simulink model "taskBlock_cursorTask_bld"  (R2012b)
settings: Solver=FixedStepDiscrete  StartTime=0.0  StopTime=10.0  FixedStep=0.001  RelTol=1e-3
undefined symbols (not defined in the file): biasCorrectionEnable, biasCorrectionInitial, biasCorrectionPower, biasCorrectionResetToInitial, biasCorrectionStateInds, biasCorrectionTau, biasCorrectionType, biasCorrectionVelocityThreshold, clickHoldTime, clickSource, gloveIndices, gloveThreshold, hmmClickLikelihoodThreshold, hmmClickSpeedMax, hmmResetOnClick, hmmResetOnFast, xkConstants
libraries: xpclib x1
settings Model: Creator=gilja  LastModifiedBy=NPTL
settings SolverCC: EnableConcurrentExecution=on  ConcurrentTasks=on
settings DataIOCC: SaveOutput=off  SignalLogging=off  SaveTime=off
settings OptimizationCC: InlineParams=on  InlineInvariantSignals=on  EnhancedBackFolding=on  EfficientFloat2IntCast=on  SimCompilerOptimization=On
settings DebuggingCC: UnderspecifiedInitializationDetection=Simplified
settings HardwareCC: ProdIntDivRoundTo=Zero  ProdEndianess=LittleEndian  ProdHWDeviceType=Generic->32-bit x86 compatible
settings ModelReferenceCC: ModelReferenceNumInstancesAllowed=Single  ModelReferenceMinAlgLoopOccurrences=on
settings RTWCC: SystemTargetFile=xpctarget.tlc  TemplateMakefile=xpc_default_tmf  Description=xPC Target  ProcessScript=xpctarget_make_rtw_hook  RTWCompilerOptimization=On
settings CodeAppCC: MaxIdLength=62
settings xpcTargetCC: TargetFcnLib=ansi_tfl_table_tmw.mat  CodeReplacementLibrary=XPC_BLAS  ParMdlRefBuildCompliant=on  ConcurrentExecutionCompliant=on  CombineSignalStateStructs=off  GRTInterface=on  xPCTaskExecutionProfile=on  xPCRL32EventNumber=5000  xPCisDownloadable=off  xPCLoadParamSetFile=off  xPCConcurrentTasks=off  xPCEnableSFAnimation=off

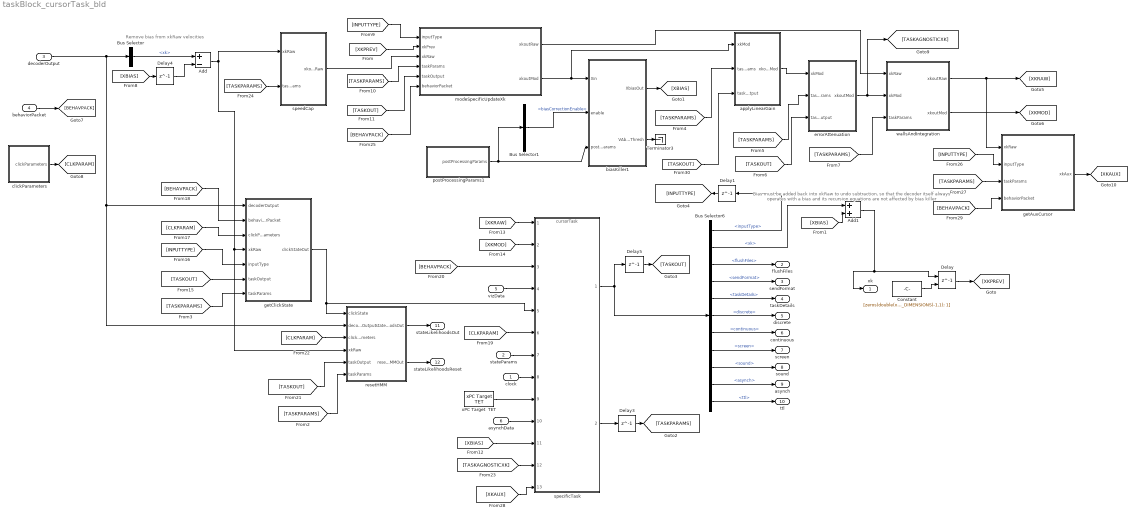
== system taskBlock_cursorTask_bld ==
  note: Remove bias from xkRaw velocities
  note: Bias must be added back into xkRaw to undo subtraction,
      | so that the decoder itself always operates with a bias and its
      | recursion equations are not affected by bias killer
  clock : Inport  OutDataTypeStr=uint32
  stateParams : Inport  Port=2  OutDataTypeStr=Bus: stateParams
  decoderOutput : Inport  Port=3  OutDataTypeStr=Bus: decoderOutput
  behaviorPacket : Inport  Port=4  OutDataTypeStr=Bus: behaviorPacketBus
  vizData : Inport  Port=5  OutDataTypeStr=Bus: peripheralData
  asynchData : Inport  Port=6  OutDataTypeStr=Bus: peripheralData
  Add : Sum  Inputs=+-
  Add1 : Sum
  Bus Selector : BusSelector  OutputSignals=xk
  Bus Selector1 : BusSelector  OutputSignals=biasCorrectionEnable
  Bus Selector6 : BusSelector  OutputSignals=inputType,xk,flushFiles,sendFormat,taskDetails,discrete,continuous,screen,sound,asynch,ttl
  Constant : Constant  Value=[zeros(double(xkConstants.NUM_STATE_DIMENSIONS)-1,1); 1]  VectorParams1D=off
  Delay : Delay  DelayLength=1  InitialConditionSource=Input port  InitialCondition=0
      settings: InputPortMap=u0,p4
  Delay{1,3..5} (4 alike) : Delay  DelayLength=1  InitialCondition=0
  Terminator3 : Terminator
  applyLinearGain : MATLAB Function  TreatAsAtomicUnit=on
  biasKiller1 : MATLAB Function  TreatAsAtomicUnit=on
  clickParameters : Subsystem
  errorAttenuation : MATLAB Function  TreatAsAtomicUnit=on
  getAuxCursor : MATLAB Function  TreatAsAtomicUnit=on
  getClickState : MATLAB Function  TreatAsAtomicUnit=on
  modeSpecificUpdateXk : MATLAB Function  TreatAsAtomicUnit=on
  postProcessingParams1 : Subsystem
  resetHMM : MATLAB Function  TreatAsAtomicUnit=on
  specificTask : ModelReference  ModelNameDialog=cursorTask  SimulationMode=Normal  ModelReferenceVersion=1.2385  CopyOfModelName=cursorTask  DefaultDataLogging=on
  speedCap : MATLAB Function  TreatAsAtomicUnit=on
  wallsAndIntegration : MATLAB Function  TreatAsAtomicUnit=on
  "xPC Target  TET " : xpclib/Misc./xPC Target  TET   ts=0.001
  xk : Outport
  flushFiles : Outport  Port=2
  sendFormat : Outport  Port=3
  taskDetails : Outport  Port=4  OutDataTypeStr=Bus: fileLoggerFormat  BusOutputAsStruct=on
  discrete : Outport  Port=5  OutDataTypeStr=Bus: fileLoggerFormatAndData  BusOutputAsStruct=on
  continuous : Outport  Port=6  OutDataTypeStr=Bus: fileLoggerFormatAndData  BusOutputAsStruct=on
  screen : Outport  Port=7  OutDataTypeStr=Bus: fileLoggerFormatAndData  BusOutputAsStruct=on
  sound : Outport  Port=8  OutDataTypeStr=Bus: fileLoggerFormatAndData  BusOutputAsStruct=on
  asynch : Outport  Port=9  OutDataTypeStr=Bus: fileLoggerFormatAndData  BusOutputAsStruct=on
  ttl : Outport  Port=10  OutDataTypeStr=double  BusOutputAsStruct=on
  stateLikelihoodsOut : Outport  Port=11  OutDataTypeStr=double  BusOutputAsStruct=on
  stateLikelihoodsReset : Outport  Port=12  OutDataTypeStr=double  PortDimensions=1  BusOutputAsStruct=on
  wires:
  specificTask/1 -> Delay5/1, Bus Selector6/1
  Bus Selector6/2 -> Add1/1  "<xk>"
  Bus Selector6/3 -> flushFiles/1  "<flushFiles>"
  Bus Selector6/4 -> sendFormat/1  "<sendFormat>"
  Bus Selector6/6 -> discrete/1  "<discrete>"
  Bus Selector6/7 -> continuous/1  "<continuous>"
  Bus Selector6/5 -> taskDetails/1  "<taskDetails>"
  Bus Selector6/8 -> screen/1  "<screen>"
  Bus Selector6/1 -> Delay1/1  "<inputType>"
  decoderOutput/1 -> resetHMM/2(decoderOutput), getClickState/1(decoderOutput), Bus Selector/1
  Add/1 -> resetHMM/4(xkRaw), getClickState/4(xkRaw), speedCap/1(xkRaw)
  Bus Selector6/11 -> ttl/1  "<ttl>"
  Bus Selector6/9 -> sound/1  "<sound>"
  Bus Selector6/10 -> asynch/1  "<asynch>"
  vizData/1 -> specificTask/4
  resetHMM/1(stateLikelihoodsOut) -> stateLikelihoodsOut/1
  resetHMM/2(resetHMMOut) -> stateLikelihoodsReset/1
  specificTask/2 -> Delay3/1
  asynchData/1 -> specificTask/10
  "xPC Target  TET "/1 -> specificTask/9
  clock/1 -> specificTask/8
  stateParams/1 -> specificTask/7
  Bus Selector/1 -> Add/1  "<xk>"
  Add1/1 -> xk/1, Delay/1
  postProcessingParams1/1(postProcessingParams) -> Bus Selector1/1, biasKiller1/3(postProcParams)
  biasKiller1/2(VAboveThresh) -> Terminator3/1
  Bus Selector1/1 -> biasKiller1/2(enable)  "<biasCorrectionEnable>"
  modeSpecificUpdateXk/2(xkoutMod) -> applyLinearGain/1(xkMod), biasKiller1/1(Xin)
  modeSpecificUpdateXk/1(xkoutRaw) -> wallsAndIntegration/1(xkRaw)
  errorAttenuation/1(xkoutMod) -> [TASKAGNOSTICXK], wallsAndIntegration/2(xkMod)
  Constant/1 -> Delay/2
  Delay/1 -> [XKPREV]
  [XKPREV] -> modeSpecificUpdateXk/2(xkPrev)
  biasKiller1/1(XbiasOut) -> [XBIAS]
  [XBIAS] -> Add1/2
  Delay3/1 -> [TASKPARAMS]
  [TASKPARAMS] -> resetHMM/6(taskParams)
  [TASKPARAMS] -> getClickState/7(taskParams)
  [TASKPARAMS] -> applyLinearGain/2(taskParams)
  [TASKPARAMS] -> errorAttenuation/2(taskParams)
  Delay5/1 -> [TASKOUT]
  [TASKOUT] -> errorAttenuation/3(taskOutput)
  [TASKPARAMS] -> wallsAndIntegration/3(taskParams)
  Delay1/1 -> [INPUTTYPE]
  [INPUTTYPE] -> modeSpecificUpdateXk/1(inputType)
  [XBIAS] -> Delay4/1
  Delay4/1 -> Add/2
  [TASKPARAMS] -> modeSpecificUpdateXk/4(taskParams)
  [TASKOUT] -> modeSpecificUpdateXk/5(taskOutput)
  [XBIAS] -> specificTask/11
  wallsAndIntegration/1(xkoutRaw) -> getAuxCursor/1(xkRaw), [XKRAW]
  wallsAndIntegration/2(xkoutMod) -> [XKMOD]
  [XKRAW] -> specificTask/1
  [XKMOD] -> specificTask/2
  getClickState/1(clickStateOut) -> specificTask/5, resetHMM/1(clickState)
  behaviorPacket/1 -> [BEHAVPACK]
  clickParameters/1(clickParameters) -> [CLKPARAM]
  [TASKOUT] -> getClickState/6(taskOutput)
  [INPUTTYPE] -> getClickState/5(inputType)
  [CLKPARAM] -> getClickState/3(clickParameters)
  [BEHAVPACK] -> getClickState/2(behaviorPacket)
  [CLKPARAM] -> specificTask/6
  [BEHAVPACK] -> specificTask/3
  [TASKOUT] -> resetHMM/5(taskOutput)
  [CLKPARAM] -> resetHMM/3(clickParameters)
  applyLinearGain/1(xkoutMod) -> errorAttenuation/1(xkMod)
  [TASKAGNOSTICXK] -> specificTask/12
  [TASKPARAMS] -> speedCap/2(taskParams)
  speedCap/1(xkoutRaw) -> modeSpecificUpdateXk/3(xkRaw)
  [BEHAVPACK] -> modeSpecificUpdateXk/6(behaviorPacket)
  [INPUTTYPE] -> getAuxCursor/2(inputType)
  [TASKPARAMS] -> getAuxCursor/3(taskParams)
  getAuxCursor/1(xkAux) -> [XKAUX]
  [XKAUX] -> specificTask/13
  [BEHAVPACK] -> getAuxCursor/4(behaviorPacket)
  [TASKOUT] -> applyLinearGain/3(taskOutput)

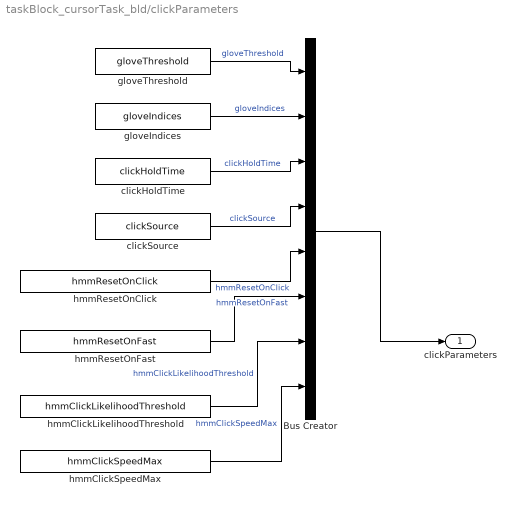
== system taskBlock_cursorTask_bld/clickParameters ==
  Bus Creator : BusCreator  Inputs='gloveThreshold','gloveIndices','clickHoldTime','clickSource','hmmResetOnClick','hmmResetOnFast','hmmClickLikelihoodThreshold','hmmClickSpeedMax'  OutDataTypeStr=Bus: clickParametersBus
  clickHoldTime : Constant  Value=clickHoldTime
  clickSource : Constant  Value=clickSource
  gloveIndices : Constant  Value=gloveIndices
  gloveThreshold : Constant  Value=gloveThreshold
  hmmClickLikelihoodThreshold : Constant  Value=hmmClickLikelihoodThreshold  VectorParams1D=off
  hmmClickSpeedMax : Constant  Value=hmmClickSpeedMax  VectorParams1D=off
  hmmResetOnClick : Constant  Value=hmmResetOnClick  VectorParams1D=off
  hmmResetOnFast : Constant  Value=hmmResetOnFast  VectorParams1D=off
  clickParameters : Outport
  wires:
  Bus Creator/1 -> clickParameters/1
  gloveThreshold/1 -> Bus Creator/1  "gloveThreshold"
  gloveIndices/1 -> Bus Creator/2  "gloveIndices"
  clickHoldTime/1 -> Bus Creator/3  "clickHoldTime"
  clickSource/1 -> Bus Creator/4  "clickSource"
  hmmResetOnClick/1 -> Bus Creator/5  "hmmResetOnClick"
  hmmClickLikelihoodThreshold/1 -> Bus Creator/7  "hmmClickLikelihoodThreshold"
  hmmClickSpeedMax/1 -> Bus Creator/8  "hmmClickSpeedMax"
  hmmResetOnFast/1 -> Bus Creator/6  "hmmResetOnFast"

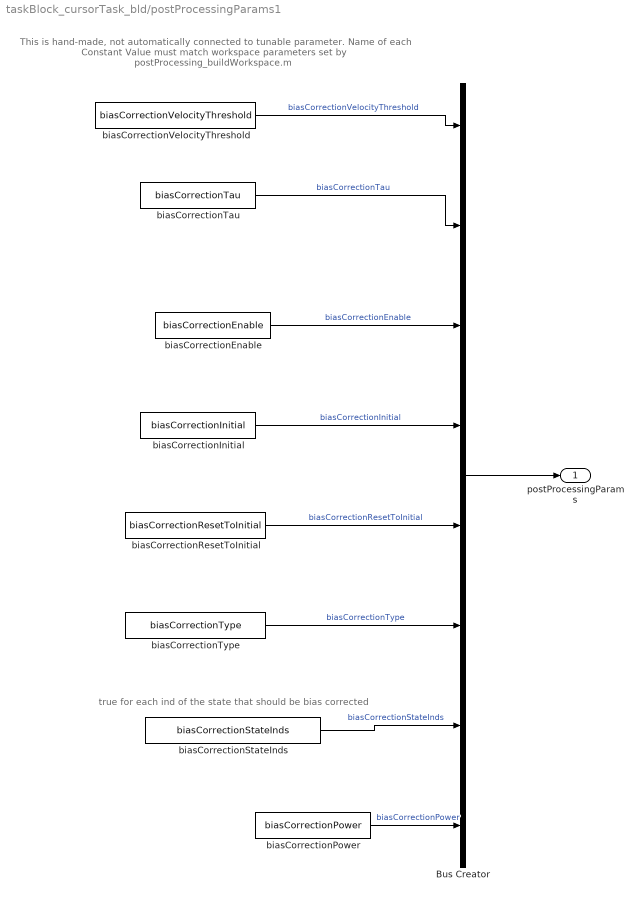
== system taskBlock_cursorTask_bld/postProcessingParams1 ==
  note: true for each ind of the state that should be bias corrected
  note: This is hand-made, not automatically connected to tunable parameter.
      | Name of each Constant Value must match workspace parameters set by
      | postProcessing_buildWorkspace.m
  Bus Creator : BusCreator  Inputs=8  OutDataTypeStr=Bus: postProcessingParams  NonVirtualBus=on
  biasCorrectionEnable : Constant  Value=biasCorrectionEnable
  biasCorrectionInitial : Constant  Value=biasCorrectionInitial
  biasCorrectionPower : Constant  Value=biasCorrectionPower
  biasCorrectionResetToInitial : Constant  Value=biasCorrectionResetToInitial
  biasCorrectionStateInds : Constant  Value=biasCorrectionStateInds
  biasCorrectionTau : Constant  Value=biasCorrectionTau
  biasCorrectionType : Constant  Value=biasCorrectionType
  biasCorrectionVelocityThreshold : Constant  Value=biasCorrectionVelocityThreshold
  postProcessingParams : Outport
  wires:
  Bus Creator/1 -> postProcessingParams/1
  biasCorrectionVelocityThreshold/1 -> Bus Creator/1  "biasCorrectionVelocityThreshold"
  biasCorrectionEnable/1 -> Bus Creator/3  "biasCorrectionEnable"
  biasCorrectionTau/1 -> Bus Creator/2  "biasCorrectionTau"
  biasCorrectionInitial/1 -> Bus Creator/4  "biasCorrectionInitial"
  biasCorrectionResetToInitial/1 -> Bus Creator/5  "biasCorrectionResetToInitial"
  biasCorrectionType/1 -> Bus Creator/6  "biasCorrectionType"
  biasCorrectionStateInds/1 -> Bus Creator/7  "biasCorrectionStateInds"
  biasCorrectionPower/1 -> Bus Creator/8  "biasCorrectionPower"

== matlab function taskBlock_cursorTask_bld/resetHMM ==
  data: clickState input; decoderOutput input Bus: decoderOutput; stateLikelihoodsOut output double; clickParameters input Bus: clickParametersBus; resetHMMOut output; xkRaw input; taskOutput input; taskParams input
function [stateLikelihoodsOut, resetHMMOut] = resetHMM(clickState, decoderOutput, clickParameters, xkRaw, taskOutput, taskParams)
%% takes in all of the state likelihoods and changes move's state likelihood to 1 and the rest to 0 if a reset is triggered
% Checks all the ways the HMM can be reset: 
%%% Exceeding the speed threshold
%%% The click time has elapsed. 
%%% The task says to (eg reset on new trial) 
% only uses the value of clickState to increment the click timer or reset 
%%% SNF warns that the "taskOutput.resetHMM" option doesn't reset the state
%%% likelihoods like the rest of the cases. just so you know. Aug 2019
%%% oh and also the switch statement is uneccessary so if we wanted the
%%% functional bits to be clumped together better, we could just take it
%%% out so it's clear that the clickTime only matters if
%%% clickParameters.hmmResetOnClick is true or the speed crap only gets
%%% calculated if clickParameters.hmmResetOnFast is true. -SNF Anyway,
%%% here's wonderwall. i mean, the code: 
%% define and initialize the persistents 
persistent clickTime; %count how long the click has been held
if isempty(clickTime) %it's the beginning so no clicks yet to count 
    clickTime = 0;
end

persistent prevClickState; %SNF multiclick - compare current click to previous
if isempty(prevClickState) %if there hasn't been a click signal yet, initialize to current clickState
    prevClickState = uint16(clickState); 
end
%% define likelihoods that will be assigned if a reset is triggered
resetLikelihoods = zeros([double(DecoderConstants.MAX_DISCRETE_STATES) 1]); 
resetLikelihoods(1) = 1; % when things are reset, move should be active and no others should be
resetHMMOut = 0; %by default, a reset hasn't been triggered
%% Reset check: has the click exceeded click time? 
%if clickState == uint16(DiscreteStates.CLICK_MAIN) % <- old version, pre-mulitclick
%SNF: increment clickTime if the current click matches the previous one, otherwise reset 
if (uint16(clickState) >= uint16(DiscreteStates.CLICK_MAIN)) % we're currently clicking
    if (prevClickState == uint16(clickState)) || (prevClickState == uint16(DiscreteStates.CLICK_IDLE)) %the previous click was this one OR idle
        clickTime = clickTime+1;
    else %transitioned from a previous click. This shouldn't ever happen but we'll write it out just in case. 
         clickTime = 0; %transitioning from a previous click directly is not allowed, treat it like IDLE  
    end    
else % clickState is IDLE, reset click time
    clickTime = 0;  
end
prevClickState = uint16(clickState); %this should always reflect the last clickState *unless a reset is triggered* (below)
%% copy stateLikelihoods from input to output
stateLikelihoodsOut = decoderOutput.stateLikelihoods;
%% calculate current speed to see if we need to reset bc of speed 
xk2HorizontalVel = uint8( taskParams.xk2HorizontalVel );
xk2VerticalVel   = uint8( taskParams.xk2VerticalVel );
xk2DepthVel      = uint8( taskParams.xk2DepthVel );
velInds          = [xk2HorizontalVel, xk2VerticalVel, xk2DepthVel];
speed            = sqrt(sum(xkRaw(velInds).^2));
%% go through our reset options to see if a reset should be triggered 
switch clickParameters.clickSource %why do we have a switch here? OL never needs this reset so... ? 
    case clickConstants.CLICK_TYPE_NEURAL %Closed loop
    %% we've reach max click time and the task says to auto release after click, reset
        if clickParameters.hmmResetOnClick && clickTime >= clickParameters.clickHoldTime 
            stateLikelihoodsOut = resetLikelihoods; %make move 1 and all others 0
            clickTime = 0;                          %reset the click clock
            resetHMMOut = 1;                        %signal the reset 
            prevClickState = uint16(DiscreteStates.CLICK_IDLE); % update the state
        end
   %% reset to 0 if we're going too fast and the task says to
        if clickParameters.hmmResetOnFast && speed > clickParameters.hmmClickSpeedMax
            stateLikelihoodsOut = resetLikelihoods; %make move 1 and all others 0
            clickTime = 0;                          %reset the click clock
            resetHMMOut = 1;                        %signal the reset 
            prevClickState = uint16(DiscreteStates.CLICK_IDLE); % update the state
        end
   %% task can reset HMM at any time
        if taskOutput.resetHMM %SNF says: WHOAAAAAA WTF why don't we reset the likelihoods here???? But also not touching that. 
            clickTime = 0;
            resetHMMOut = 1;
        end
end %nevermind that this switch statement is useless and is throwing off the groove of the rest of the code.

== matlab function taskBlock_cursorTask_bld/speedCap ==
  data: xkRaw input; xkoutRaw output size=[double(xkConstants.NUM_STATE_DIMENSIONS),1]; taskParams input
function xkoutRaw  = applySpeedCap(xkRaw, taskParams)

%applies speed cap, using the cap in taskParams.xkRawSpeedCap
NUM_DIMS = uint8(cursorConstants.NUM_DIMENSIONS); 
xk2HorizontalVel = uint8( taskParams.xk2HorizontalVel );
xk2VerticalVel = uint8( taskParams.xk2VerticalVel );
xk2DepthVel = uint8( taskParams.xk2DepthVel );
xk2RotateVel = uint8( taskParams.xk2RotateVel );
xk2Rotate2Vel = uint8( taskParams.xk2Rotate2Vel );

canBeVelInds = [xk2HorizontalVel,xk2VerticalVel,xk2DepthVel,xk2RotateVel,xk2Rotate2Vel];
effectorVelInds = canBeVelInds(1:NUM_DIMS);

xkoutRaw = xkRaw;
currentSpeed = sqrt(sum(xkRaw(effectorVelInds).^2)) + eps;
if currentSpeed > taskParams.xkRawSpeedCap
    newSpeed = double(taskParams.xkRawSpeedCap);
else
    newSpeed = currentSpeed;
end
xkoutRaw(effectorVelInds) = xkoutRaw(effectorVelInds) * (newSpeed / currentSpeed);

end

== matlab function taskBlock_cursorTask_bld/biasKiller1 ==
  data: Xin input; enable input; postProcParams input; XbiasOut output; VAboveThresh output
function [XbiasOut, VAboveThresh] = biasKiller(Xin, enable, postProcParams)


speedThreshold = postProcParams.biasCorrectionVelocityThreshold;
tau = postProcParams.biasCorrectionTau;
biasCorrectionInitial = postProcParams.biasCorrectionInitial;
biasCorrectionResetToInitial = postProcParams.biasCorrectionResetToInitial;
biasCorrectionType = postProcParams.biasCorrectionType;
biasCorrectionPower =  postProcParams.biasCorrectionPower; % for BIAS_CORRECTION_SERGEY

% bcInds = postProcParams.biasCorrectionStateInds; % Which elements of state are tracked SDS 7/2016
bcInds = [2:2:20]; %SDS/BJ: should be all the velocity indices of kinematic state

persistent Xbias;
if isempty(Xbias)
    Xbias = zeros(size(Xin));
end
if biasCorrectionResetToInitial
    Xbias = biasCorrectionInitial;
end

VAboveThresh = false;

if enable && tau > 0
    % if tau > 0 update the bias estimate. Setting tau to 0 locks the bias
    % estimate down at whatever it previously was. 
    speed = sqrt( sum( (double(Xin(bcInds))).^2 ) ); %    speed must be greater than some threshold.
 
    switch biasCorrectionType
        % squares each dimension before accumulating it into bias estimate
        case DecoderConstants.BIAS_CORRECTION_FRANK  %% Frank's unbiased killer            
            if (double(speed) > double(speedThreshold))
                Xbias(bcInds) = Xbias(bcInds) + double(Xin(bcInds)) .* abs(double(Xin(bcInds))) ./ double(tau);
                VAboveThresh = true;
            end
            
        case DecoderConstants.BIAS_CORRECTION_BEATA
             % linearly adds each dimension before accumulating it into bias estimate
            if (double(speed) > double(speedThreshold))
                Xbias(bcInds) = Xbias(bcInds) + double(Xin(bcInds)) ./ double(tau);
                VAboveThresh = true;
            end
            
        case DecoderConstants.BIAS_CORRECTION_SERGEY
            % normalizes high-D speed to threshold, then squares, then reverses normalization, then accumulates
            if (double(speed) > double(speedThreshold))                
                normFactor = 1 / double( speedThreshold );
                VinScaled = normFactor .* double( Xin(bcInds) ); % decoded velocity, scaled to >1 by normalizing to speedThreshold
                Vweight = norm( VinScaled ) .^ biasCorrectionPower; % to the power of <biasCorrectionPower> is the scaling rate; so faster speeds weighted  more
                biasUpdate = double(Xin(bcInds)) .* Vweight; % scaled
                biasUpdate = biasUpdate ./ double( tau ); % larger tau slows down bias accumulation.
                Xbias(bcInds) = Xbias(bcInds) + biasUpdate;
                
                VAboveThresh = true;
            end
    end
elseif enable && tau == 0
    % if tau == 0 don't worry about adapting / updating the bias estimate
else
    Xbias = zeros(size(Xin));
end

XbiasOut = Xbias;

== matlab function taskBlock_cursorTask_bld/modeSpecificUpdateXk ==
  data: inputType input uint16 size=1; xkPrev input size=[double(xkConstants.NUM_STATE_DIMENSIONS),1]; xkRaw input size=[double(xkConstants.NUM_STATE_DIMENSIONS),1]; xkoutRaw output size=[double(xkConstants.NUM_STATE_DIMENSIONS),1]; taskParams input; taskOutput input; xkoutMod output size=[double(xkConstants.NUM_STATE_DIMENSIONS),1]; behaviorPacket input
function [xkoutRaw, xkoutMod] = modeSpecificUpdateXk(inputType, xkPrev, xkRaw, taskParams, taskOutput, behaviorPacket)
% xkoutRaw is destined for being fed back into the decoder. 
%xkoutMod ("modified") will affect the task but will not be fed back to the
%decoder. Things like error attenuation should happen to it so that they
%are not compounded by the decoder.

% Most of these persistent variables are used for autoplay (some also for
% error assist). When introducing rotation DOF, I want the autoplay to do
% these rotations *after* the translation. So now there is an additional
% time endpoint (timeFinalRot) 
% -SDS Feb 22 2017
persistent xkStart xTgt prevState timeFinal time timeFinalRot;

NUM_DIMS = uint8(cursorConstants.NUM_DIMENSIONS); % dimensionality of the task. Fixed for a given compile

if(isempty(xkStart))
    xkStart = xkPrev;
    prevState = uint16(0); %% was - uint16(CursorStates.STATE_INIT), this leads to conflicts;
    xTgt = double(zeros(NUM_DIMS,1)); % vector t the target
    timeFinal = 0; % Translation end time.
    timeFinalRot = 0; % Rotation end time. Note that rotation starts after timeFinal + autoplayReactionTime
    time = 0; %will be used to keep track of ti
end

% which state elements do I look to for relevant kinematics pos/vel?
xk2HorizontalPos = uint8( taskParams.xk2HorizontalPos );
xk2VerticalPos = uint8( taskParams.xk2VerticalPos );
xk2HorizontalVel = uint8( taskParams.xk2HorizontalVel );
xk2VerticalVel = uint8( taskParams.xk2VerticalVel );
xk2DepthPos = uint8( taskParams.xk2DepthPos );
xk2DepthVel = uint8( taskParams.xk2DepthVel );
xk2RotatePos = uint8( taskParams.xk2RotatePos );
xk2RotateVel = uint8( taskParams.xk2RotateVel );
xk2Rotate2Pos = uint8( taskParams.xk2Rotate2Pos );
xk2Rotate2Vel = uint8( taskParams.xk2Rotate2Vel );
% DIMENSION-DEPENDENT

canBePosInds = [xk2HorizontalPos,xk2VerticalPos,xk2DepthPos,xk2RotatePos,xk2Rotate2Pos];
effectorPosInds = canBePosInds(1:NUM_DIMS);
canBeVelInds = [xk2HorizontalVel,xk2VerticalVel,xk2DepthVel,xk2RotateVel,xk2Rotate2Vel];
effectorVelInds = canBeVelInds(1:NUM_DIMS);

% Which are translation and which are rotation dimensions?
if NUM_DIMS > 3 % might need to be updated if we add an aperture or other type of DOF later
    NUM_TRANS_DIMS = 3;
    effectorTransPosInds = effectorPosInds(1:NUM_TRANS_DIMS);
    effectorRotPosInds = effectorPosInds(NUM_TRANS_DIMS+1:NUM_DIMS);
    effectorTransVelInds = effectorVelInds(1:NUM_TRANS_DIMS);
    effectorRotVelInds = effectorVelInds(NUM_TRANS_DIMS+1:NUM_DIMS);
    % DIMENSION-DEPENDENT [only if going beyond just rotational dims)
else
    effectorTransPosInds = effectorPosInds;
    effectorRotPosInds = [];
    effectorTransVelInds = effectorVelInds;
    effectorRotVelInds = [];
    NUM_TRANS_DIMS = NUM_DIMS;
end

% SDS October 31 2016
% make last element of xk 1 here. it used to happen in the specificTask,
% which doesn't make sense. Note that we also set this again in the
% decoder, which is redundant, but there it's there just in case we don't
% do it here, and ehre we do it so that this gets logged in
% stream.continuous.xk (since the decoderOutput.xk is different).
xkPrev(end) = 1;

xkoutRaw = xkPrev;

% Set all velocity states to zero. Assumption is that velocity  
% are even indices. These get filled in with modified velocities later in
% this block.
xkoutRaw(2:2:size(xkoutRaw,1)-1) = 0;

% start by making xkoutMod equal to xkoutRaw
xkoutMod = xkoutRaw;

% SDS May 2 2017: Removed logic which checks whether to stop cursor upon a
% click. This is because it was not taking clickHoldTime into account, such
% that a brief click would cause stopping. That's too sensitive.
% Integrating click state to determine selection or velocity zeroing will
% now be relegated to the specificTask.

autoacquireMoveStates = double([CursorStates.STATE_MOVE CursorStates.STATE_MOVE_CLICK CursorStates.STATE_CENTER_TARGET CursorStates.STATE_ACQUIRE CursorStates.STATE_HOVER]);

switch inputType
    case {cursorConstants.INPUT_TYPE_DECODE_V, cursorConstants.INPUT_TYPE_HEAD_CURSORSTILL, ...
            cursorConstants.INPUT_TYPE_CURSOR_HEADSTILL, cursorConstants.INPUT_TYPE_CURSOR_AND_HEAD} 
        % Neural decode -- most common use case
        % Puts this model tick's decoder output into the velocity
        xkoutRaw(effectorVelInds) = xkRaw(effectorVelInds);
        xkoutMod(effectorVelInds) = xkRaw(effectorVelInds);
        
        % Nonlinear gain.
        % applies a nonlinear power gain, which is governed by
        % two parameters. the powerGain determines the shape
        % of the curve (higher values have a steeper rise).
        % The powerGainUnityCrossing defines the superlinear cross-over point
        % after which the output equals the input. - SDS April 2017
        inSpeed = sqrt( sum(  xkoutMod(effectorVelInds).^2 ) );
        inScaled =  inSpeed./ taskParams.powerGainUnityCrossing; % speed, as a multiple of unity crossing
        outScaled = inScaled ^ taskParams.powerGain; % how much slower/faster it got
        if inSpeed < eps
            % avoids nans when divide by 0 would happen
            unitNormVel =  xkoutMod(effectorVelInds);
        else
            unitNormVel =  xkoutMod(effectorVelInds) ./ inSpeed;
        end
        xkoutMod(effectorVelInds) = (outScaled*taskParams.powerGainUnityCrossing) .* unitNormVel;

    case {cursorConstants.INPUT_TYPE_AUTO_ACQUIRE, cursorConstants.INPUT_TYPE_AUTO_ACQUIRE_HS, cursorConstants.INPUT_TYPE_WIA_HEAD} % ASSUMES CENTER OUT (AND BACK) WITH A SINGLE FIXED TGT DISTANCE
        if( ((prevState ~= CursorStates.STATE_MOVE) && (taskOutput.state == CursorStates.STATE_MOVE)) ...
                || ((prevState ~= CursorStates.STATE_MOVE_CLICK) && (taskOutput.state == CursorStates.STATE_MOVE_CLICK)) ...
                || ((prevState ~= CursorStates.STATE_CENTER_TARGET) && taskOutput.state == CursorStates.STATE_CENTER_TARGET))
            % game just entered one of the autoplay states, so compute
            % the vector towards the target and how long it should take
            % to get there.
            xkStart = xkPrev;
            xTgt = double(taskOutput.currentTarget(1:NUM_DIMS)) - ...
                double(xkPrev(effectorPosInds));
            
            % When translation ends: 1 autoplayReactionTime added
            if taskOutput.wiaCode==1
                speedMultiplier = 1;
                if taskOutput.speedCode==1
                    speedMultiplier = 3;
                elseif taskOutput.speedCode==2
                    speedMultiplier = 1.5;
                elseif taskOutput.speedCode==3
                    speedMultiplier = 0.75;
                end
                timeMultiplier = speedMultiplier * log(sqrt(sum(xTgt.^2)))/6.0137;
            else
                timeMultiplier = 1;
            end
            
            timeFinal = round( timeMultiplier * double( taskParams.autoplayReactionTime + taskParams.autoplayMovementDuration ) );
            
            % When rotation ends: it starts 1
            % autoplayReactionTime *after* translation ends
            timeFinalRot = round( double( taskParams.autoplayRotationStart + taskParams.autoplayRotationDuration ) );
            
            time = 0;
        elseif any(double(taskOutput.state) == autoacquireMoveStates)
            % what fraction of the translation is complete (from 0
            % to 1):
            transStartsAt = double( taskParams.autoplayReactionTime );
            tau = min( max(0, time - transStartsAt)/(timeFinal-transStartsAt), 1); % this is what it was before I fixed this on July 12 2017 -SDS
            
            % What fraction of the rotation is complete( from 0 to
            % 1)
            rotStartsAt = double( taskParams.autoplayRotationStart);
            tauRot = min( max(0, time - rotStartsAt)/(timeFinalRot-rotStartsAt) , 1); 
            
            % do this to both raw and modified. I'm not sure if we
            % actually do anything with the raw xk during filter
            % building but might as well keep behavior consistent
            % with how it was before we separated xkoutRaw and
            % xkoutMod.
            % Old way, before breaking out translation and rotation
            %                     xkoutRaw(effectorPosInds) = xkStart(effectorPosInds(1:NUM_DIMS)) -  xTgt(1:NUM_DIMS)* double( (15*tau^4 - 6*tau^5 - 10*tau^3) ); % 1:NUM_DIMS to handhold compiler
            %                     xkoutRaw(effectorVelInds) = xkoutRaw(effectorPosInds) - xkPrev(effectorPosInds);
            %                     xkoutMod(effectorPosInds) = xkoutRaw(effectorPosInds);
            %                     xkoutMod(effectorVelInds) = xkoutRaw(effectorVelInds);
            % TRANSLATION
            xkoutRaw(effectorTransPosInds) = xkStart(effectorTransPosInds) -  xTgt(1:NUM_TRANS_DIMS)* double( (15*tau^4 - 6*tau^5 - 10*tau^3) );
            xkoutRaw(effectorTransVelInds) = xkoutRaw(effectorTransPosInds) - xkPrev(effectorTransPosInds);
            xkoutMod(effectorTransPosInds) = xkoutRaw(effectorTransPosInds);
            xkoutMod(effectorTransVelInds) = xkoutRaw(effectorTransVelInds);
            
            % ROTATION
            xkoutRaw(effectorRotPosInds) = xkStart(effectorRotPosInds) -  xTgt(NUM_TRANS_DIMS+1:NUM_DIMS)* double( (15*tauRot^4 - 6*tauRot^5 - 10*tauRot^3) );
            xkoutRaw(effectorRotVelInds) = xkoutRaw(effectorRotPosInds) - xkPrev(effectorRotPosInds);
            xkoutMod(effectorRotPosInds) = xkoutRaw(effectorRotPosInds);
            xkoutMod(effectorRotVelInds) = xkoutRaw(effectorRotVelInds);
            
            time = time + 1; % time since this autoplay began counts up..
        else
            xkoutRaw(effectorVelInds) = 0;
            xkoutMod(effectorVelInds) = 0;
        end
        
    case cursorConstants.INPUT_TYPE_NONE
        xkoutRaw(effectorVelInds) = 0;
        xkoutMod(effectorVelInds) = 0;
        
    case cursorConstants.INPUT_TYPE_HEAD_MOUSE
        xkoutRaw(effectorPosInds(1)) = behaviorPacket.windowsMousePosition(1)*1080;
        xkoutRaw(effectorPosInds(2)) = -behaviorPacket.windowsMousePosition(2)*1080;
        
        xkoutMod(effectorPosInds(1)) = behaviorPacket.windowsMousePosition(1)*1080;
        xkoutMod(effectorPosInds(2)) = -behaviorPacket.windowsMousePosition(2)*1080;
        
        R = [cosd(taskParams.vmrTheta), -sind(taskParams.vmrTheta); sind(taskParams.vmrTheta), cosd(taskParams.vmrTheta)]; 
        xkoutMod(effectorPosInds(1:2)) = R*xkoutMod(effectorPosInds(1:2));
        
        xkoutRaw(effectorVelInds) = 0;
        xkoutMod(effectorVelInds) = 0;
        
    otherwise
        xkoutRaw(effectorVelInds) = 0;
        xkoutMod(effectorVelInds) = 0;
end

%for autoplay
prevState = uint16(taskOutput.state);

end

== matlab function taskBlock_cursorTask_bld/applyLinearGain ==
  data: xkMod input; xkoutMod output size=[double(xkConstants.NUM_STATE_DIMENSIONS),1]; taskParams input; taskOutput input
function xkoutMod  = applyLinearGain(xkMod, taskParams, taskOutput)

%applies linear gains to each dimension as specified in taskParams
NUM_DIMS = uint8(cursorConstants.NUM_DIMENSIONS); 
xk2HorizontalVel = uint8( taskParams.xk2HorizontalVel );
xk2VerticalVel = uint8( taskParams.xk2VerticalVel );
xk2DepthVel = uint8( taskParams.xk2DepthVel );
xk2RotateVel = uint8( taskParams.xk2RotateVel );
xk2Rotate2Vel = uint8( taskParams.xk2Rotate2Vel );

canBeVelInds = [xk2HorizontalVel,xk2VerticalVel,xk2DepthVel,xk2RotateVel,xk2Rotate2Vel];
effectorVelInds = canBeVelInds(1:NUM_DIMS);

xkoutMod = xkMod;
xkoutMod(effectorVelInds) = xkMod(effectorVelInds) .* taskParams.gain(1:NUM_DIMS,1);
if uint16(taskOutput.state) == CursorStates.STATE_NEW_TARGET
    xkoutMod(effectorVelInds) = xkoutMod(effectorVelInds) .* taskParams.delayPeriodGainScale;
end
end

== matlab function taskBlock_cursorTask_bld/wallsAndIntegration ==
  data: xkRaw input; xkMod input size=[double(xkConstants.NUM_STATE_DIMENSIONS),1]; xkoutRaw output size=[double(xkConstants.NUM_STATE_DIMENSIONS),1]; taskParams input; xkoutMod output size=[double(xkConstants.NUM_STATE_DIMENSIONS),1]
function [xkoutRaw, xkoutMod] = wallsAndIntegration(xkRaw, xkMod, taskParams)
% xkoutRaw is destined for being fed back into the decoder. 
%xkoutMod ("modified") will affect the task but will not be fed back to the
%decoder. Things like error attenuation should happen to it so that they
%are not compounded by the decoder.

NUM_DIMS = uint8(cursorConstants.NUM_DIMENSIONS); % dimensionality of the task. Fixed for a given compile

% which state elements do I look to for relevant kinematics pos/vel?
xk2HorizontalPos = uint8( taskParams.xk2HorizontalPos );
xk2VerticalPos = uint8( taskParams.xk2VerticalPos );
xk2HorizontalVel = uint8( taskParams.xk2HorizontalVel );
xk2VerticalVel = uint8( taskParams.xk2VerticalVel );
xk2DepthPos = uint8( taskParams.xk2DepthPos );
xk2DepthVel = uint8( taskParams.xk2DepthVel );
xk2RotatePos = uint8( taskParams.xk2RotatePos );
xk2RotateVel = uint8( taskParams.xk2RotateVel );
xk2Rotate2Pos = uint8( taskParams.xk2Rotate2Pos );
xk2Rotate2Vel = uint8( taskParams.xk2Rotate2Vel );

canBePosInds = [xk2HorizontalPos,xk2VerticalPos,xk2DepthPos,xk2RotatePos,xk2Rotate2Pos];
effectorPosInds = canBePosInds(1:NUM_DIMS);
canBeVelInds = [xk2HorizontalVel,xk2VerticalVel,xk2DepthVel,xk2RotateVel,xk2Rotate2Vel];
effectorVelInds = canBeVelInds(1:NUM_DIMS);

xkoutRaw = xkRaw;
xkoutMod = xkMod;

%% integrates velocity into change of position (important, obviously)
%R = [cosd(taskParams.vmrTheta), -sind(taskParams.vmrTheta); sind(taskParams.vmrTheta), cosd(taskParams.vmrTheta)]; 
%xkoutMod(effectorVelInds(1:2)) = R*xkoutMod(effectorVelInds(1:2));
 
xkoutRaw(effectorPosInds) = xkoutRaw(effectorPosInds) + xkoutRaw(effectorVelInds);
xkoutMod(effectorPosInds) = xkoutMod(effectorPosInds) + xkoutMod(effectorVelInds);

%% Boundaries to workspace
% Horizontal
if xkoutMod(taskParams.xk2HorizontalPos) > taskParams.workspaceX(2)
    xkoutMod(taskParams.xk2HorizontalPos) = taskParams.workspaceX(2);
    xkoutMod(taskParams.xk2HorizontalVel) = 0;
elseif xkoutMod(taskParams.xk2HorizontalPos) < taskParams.workspaceX(1)
    xkoutMod(taskParams.xk2HorizontalPos) = taskParams.workspaceX(1);
    xkoutMod(taskParams.xk2HorizontalVel) = 0;
end
% Vertical
if xkoutMod(taskParams.xk2VerticalPos) > taskParams.workspaceY(2)
    xkoutMod(taskParams.xk2VerticalPos) = taskParams.workspaceY(2);
    xkoutMod(taskParams.xk2VerticalVel) = 0;
elseif xkoutMod(taskParams.xk2VerticalPos) < taskParams.workspaceY(1)
    xkoutMod(taskParams.xk2VerticalPos) = taskParams.workspaceY(1);
    xkoutMod(taskParams.xk2VerticalVel) = 0;
end
% Depth
if xkoutMod(taskParams.xk2DepthPos) > taskParams.workspaceZ(2)
    xkoutMod(taskParams.xk2DepthPos) = taskParams.workspaceZ(2);
    xkoutMod(taskParams.xk2DepthVel) = 0;
elseif xkoutMod(taskParams.xk2DepthPos) < taskParams.workspaceZ(1)
    xkoutMod(taskParams.xk2DepthPos) = taskParams.workspaceZ(1);
    xkoutMod(taskParams.xk2DepthVel) = 0;
end
% Rotate 1 (around the Z axis)
if xkoutMod(taskParams.xk2RotatePos) > taskParams.workspaceR(2)
    xkoutMod(taskParams.xk2RotatePos) = taskParams.workspaceR(2);
    xkoutMod(taskParams.xk2RotateVel) = 0;
elseif xkoutMod(taskParams.xk2RotatePos) < taskParams.workspaceR(1)
    xkoutMod(taskParams.xk2RotatePos) = taskParams.workspaceR(1);
    xkoutMod(taskParams.xk2RotateVel) = 0;
end
% Rotate 2 (around the Y axis)
if xkoutMod(taskParams.xk2Rotate2Pos) > taskParams.workspaceR2(2)
    xkoutMod(taskParams.xk2Rotate2Pos) = taskParams.workspaceR2(2);
    xkoutMod(taskParams.xk2Rotate2Vel) = 0;
elseif xkoutMod(taskParams.xk2Rotate2Pos) < taskParams.workspaceR2(1)
    xkoutMod(taskParams.xk2Rotate2Pos) = taskParams.workspaceR2(1);
    xkoutMod(taskParams.xk2Rotate2Vel) = 0;
end

% DIMENSION-DEPENDENT
% xkoutRaw's positions should always match xkoutMod's positions, so
% decoder knows displayed cursor position.
xkoutRaw(effectorPosInds) =  xkoutMod(effectorPosInds);

end

== matlab function taskBlock_cursorTask_bld/errorAttenuation ==
  data: xkMod input; taskParams input; taskOutput input; xkoutMod output size=[double(xkConstants.NUM_STATE_DIMENSIONS),1]
function xkoutMod   = errorAttenuation(xkMod, taskParams, taskOutput)
% xkoutRaw is destined for being fed back into the decoder. 
%xkoutMod ("modified") will affect the task but will not be fed back to the
%decoder. Things like error attenuation should happen to it so that they
%are not compounded by the decoder.

% Most of these persistent variables are used for autoplay (some also for
% error assist). When introducing rotation DOF, I want the autoplay to do
% these rotations *after* the translation. So now there is an additional
% time endpoint (timeFinalRot) 
% -SDS Feb 22 2017

NUM_DIMS = uint8(cursorConstants.NUM_DIMENSIONS); % dimensionality of the task. Fixed for a given compile

% which state elements do I look to for relevant kinematics pos/vel?
xk2HorizontalPos = uint8( taskParams.xk2HorizontalPos );
xk2VerticalPos = uint8( taskParams.xk2VerticalPos );
xk2HorizontalVel = uint8( taskParams.xk2HorizontalVel );
xk2VerticalVel = uint8( taskParams.xk2VerticalVel );
xk2DepthPos = uint8( taskParams.xk2DepthPos );
xk2DepthVel = uint8( taskParams.xk2DepthVel );
xk2RotatePos = uint8( taskParams.xk2RotatePos );
xk2RotateVel = uint8( taskParams.xk2RotateVel );
xk2Rotate2Pos = uint8( taskParams.xk2Rotate2Pos );
xk2Rotate2Vel = uint8( taskParams.xk2Rotate2Vel );

canBePosInds = [xk2HorizontalPos,xk2VerticalPos,xk2DepthPos,xk2RotatePos,xk2Rotate2Pos];
effectorPosInds = canBePosInds(1:NUM_DIMS);
canBeVelInds = [xk2HorizontalVel,xk2VerticalVel,xk2DepthVel,xk2RotateVel,xk2Rotate2Vel];
effectorVelInds = canBeVelInds(1:NUM_DIMS);

%% apply assist if specified in taskParams
% only apply when task is unpaused
xkoutMod = xkMod;
if isfield(taskParams,'errorAssistTheta') && ~taskOutput.paused % because some tasks might not have error assist
    errorAssistTheta = double( taskParams.errorAssistTheta(1:NUM_DIMS) );     %BJ: should now be a vector (one value for each dimension in NUM_DIMS)
    errorAssistR = double( taskParams.errorAssistR(1:NUM_DIMS) );             %BJ: should now be a vector (one value for each dimension in NUM_DIMS)
    errorAssistAxis = double( taskParams.errorAssistAxis(1:NUM_DIMS) );          %Added by SDS Oct 2016
    
    % start with modified xk, which may have had gain applied to it.
    xkVel = xkoutMod(effectorVelInds);                             %BJ: current decoded cursor velocity
    xT = double(taskOutput.currentTarget(1:NUM_DIMS)) - double(xkMod(effectorPosInds)); %BJ: cursor pos to target pos vector
    
    if sum( abs(xT) < 0.001 ) == NUM_DIMS   %BJ: if cursor is within 1 mm of target in every dimension,
        %skip rest of steps in EA, rather than error-assisting
    else
        %BJ: apply error assist
        xNormT = xT ./ sqrt(sum(xT.^2));    %BJ: xNormT is normalized xT, points towards target
        projT_sc = dot(xkVel, xNormT);        %BJ: scalar projection of xkVel on xT
        projT = double( zeros( 1, NUM_DIMS ) ); % initialize
        squashVelFactor = double( zeros( 1, NUM_DIMS ) ); % initialize
        
        %BJ: apply magnitude (Rho) assist only if projection is negative
        if projT_sc < 0 % if decoded velocity was poiting away from target...
            % ... Reduce the speed according to errorAssistR, up to
            % just not allowing any movement.
            projT = projT_sc*(1-errorAssistR);   %BJ: changes the projT that gets added to the decoded velocity...
            squashVelFactor = 1 - errorAssistR;     %... and squashes the output velocity if going in wrong direction
        else
            % This happens if we're headed towards target
            projT(1:NUM_DIMS) = projT_sc;   %BJ: still need to copy projT_sc into each dimension
            squashVelFactor(1:NUM_DIMS) = 1;            %BJ: leave velocity the same
        end
        % apply error correction to modified xk
        xkoutMod(effectorVelInds) = projT.*errorAssistTheta.*xNormT' + squashVelFactor.*(1 - errorAssistTheta).*xkVel';
        
        % errorAssistAxis operates last. This will reduce the velocity
        % along every cardinal axis between 0 and 1 if and only if the
        % velocity along this axis is away from the target's coordinate
        % This looks at the final velocity *after* errorAssistTheta and
        % errorAssistR were used. Though, honestly, I haven't thought
        % through the case when one would use both errorAssistR and
        % check which
        modDims = sign(xkoutMod(effectorVelInds).*xT) < 0; % 1s for any axis it's moving the wrong way at.
        % errorAssistAxis == 0 means do nothing, hence 1-__
        xkoutMod(effectorVelInds(modDims)) = xkoutMod(effectorVelInds(modDims)).*(1-errorAssistAxis(modDims))';
    end
end

end

== matlab function taskBlock_cursorTask_bld/getAuxCursor ==
  data: xkRaw input; inputType input; xkAux output size=[double(xkConstants.NUM_STATE_DIMENSIONS),1]; taskParams input; behaviorPacket input
function xkAux = getAuxCursor(xkRaw, inputType, taskParams, behaviorPacket)
    %Some modes have an extra "auxiliary" cursor (e.g. when the head mouse cursor must be
    %held still while the BCI cursor must acquire targets as normal). Based on the mode, this block
    %outputs the auxiliary cursor state. Right now it works only for the head
    %mouse. 

    NUM_DIMS = uint8(cursorConstants.NUM_DIMENSIONS); 

    xk2HorizontalPos = uint8( taskParams.xk2HorizontalPos );
    xk2VerticalPos = uint8( taskParams.xk2VerticalPos );
    xk2HorizontalVel = uint8( taskParams.xk2HorizontalVel );
    xk2VerticalVel = uint8( taskParams.xk2VerticalVel );
    xk2DepthPos = uint8( taskParams.xk2DepthPos );
    xk2DepthVel = uint8( taskParams.xk2DepthVel );
    xk2RotatePos = uint8( taskParams.xk2RotatePos );
    xk2RotateVel = uint8( taskParams.xk2RotateVel );
    xk2Rotate2Pos = uint8( taskParams.xk2Rotate2Pos );
    xk2Rotate2Vel = uint8( taskParams.xk2Rotate2Vel );

    canBePosInds = [xk2HorizontalPos,xk2VerticalPos,xk2DepthPos,xk2RotatePos,xk2Rotate2Pos];
    effectorPosInds = canBePosInds(1:NUM_DIMS);
    canBeVelInds = [xk2HorizontalVel,xk2VerticalVel,xk2DepthVel,xk2RotateVel,xk2Rotate2Vel];
    effectorVelInds = canBeVelInds(1:NUM_DIMS);

    xkAux = zeros(size(xkRaw));

    switch inputType
        case {cursorConstants.INPUT_TYPE_HEAD_CURSORSTILL, cursorConstants.INPUT_TYPE_CURSOR_HEADSTILL, ...
                cursorConstants.INPUT_TYPE_AUTO_ACQUIRE_HS, cursorConstants.INPUT_TYPE_CURSOR_AND_HEAD, cursorConstants.INPUT_TYPE_WIA_HEAD}
            xkAux(effectorPosInds(1)) = behaviorPacket.windowsMousePosition(1)*1080;
            xkAux(effectorPosInds(2)) = -behaviorPacket.windowsMousePosition(2)*1080;
            xkAux(effectorVelInds) = 0;

        otherwise
            xkAux(effectorVelInds) = 0;
            xkAux(effectorVelInds) = 0; 
    end
end

== matlab function taskBlock_cursorTask_bld/getClickState ==
  data: decoderOutput input; behaviorPacket input Bus: behaviorPacketBus; clickStateOut output uint16; clickParameters input Bus: clickParametersBus; xkRaw input; inputType input; taskOutput input; taskParams input
function clickStateOut = getClickState(decoderOutput, behaviorPacket, clickParameters, xkRaw, inputType, taskOutput, taskParams)
% clickStateOut ranges from IDLE to any of the clicks (multiclick) -
% identify it based on the state likelihoods in decoderOutput and
% clickParameters (for the threshold). This block takes the decoded output
% and does the deciding so the task only gets the decoded click value. 
% -last modified and commented by SNF, August 2019 
% the xk here is xkRaw 
%% define the (unecessary) persistent. SNF can't spell unnecessary and she knows. uneccessary? *shrugs*
% SNF: this initialization is uneccessary, also doesn't need to be persistent since we
% always set it to idle at the beginning.... 
%  persistent clickState ;
% if isempty(clickState)
%     clickState = uint16(DiscreteStates.CLICK_IDLE);
% end
clickState = uint16(DiscreteStates.CLICK_IDLE); %SNF: this line was already here, outside of the if so yeah no persistence necessary
%% get the cursor position (- but really the velocity is all that matters -SNF) 
% which state elements do I look to for the cursor's position? SDS July 2016
NUM_DIMS         = uint8(cursorConstants.NUM_DIMENSIONS); % 
xk2HorizontalPos = uint8( taskParams.xk2HorizontalPos );
xk2VerticalPos   = uint8( taskParams.xk2VerticalPos );
xk2HorizontalVel = uint8( taskParams.xk2HorizontalVel );
xk2VerticalVel   = uint8( taskParams.xk2VerticalVel );
xk2DepthPos      = uint8( taskParams.xk2DepthPos );
xk2DepthVel      = uint8( taskParams.xk2DepthVel );
xk2RotatePos     = uint8( taskParams.xk2RotatePos );
xk2RotateVel     = uint8( taskParams.xk2RotateVel );
xk2Rotate2Pos    = uint8( taskParams.xk2Rotate2Pos );
xk2Rotate2Vel    = uint8( taskParams.xk2Rotate2Vel );
% TASK_DIMS = taskParams.numDisplayDims; % only used for determining what kind of
% % checking to use. We still need to have everything be NUM_DIMS long or things won't compile.
canBePosInds = [xk2HorizontalPos,xk2VerticalPos,xk2DepthPos,xk2RotatePos,xk2Rotate2Pos];
canBeVelInds = [xk2HorizontalVel,xk2VerticalVel,xk2DepthVel,xk2RotateVel,xk2Rotate2Vel];
effectorPosInds = canBePosInds(1:NUM_DIMS);
effectorVelInds = canBeVelInds(1:NUM_DIMS);
% and get the speed while we're here
speed = sqrt(sum(xkRaw(effectorVelInds).^2));
%% initialize multiclick variables 
CLICK_INDICES = 2: uint16(DecoderConstants.MAX_DISCRETE_STATES);
maxCS  = double(0); % there is some CRAZY type casting necessary for Simulink, don't mind this.... 
maxL   = double(0);
%% handle ancient artifacts: 
gloveData = behaviorPacket.glove;
if behaviorPacket.gloveSerial2(6) == 'L'
    gloveData = behaviorPacket.glove2;
end
% less ancient, still old and unused: 
mouseData = behaviorPacket.mouse;
%% assign clickState values!
if inputType == cursorConstants.INPUT_TYPE_AUTO_ACQUIRE % OL is so easy 
    if taskOutput.state == CursorStates.STATE_HOVER     % if it's an instructed click target
        % original: this is now the else clause 
%              clickState = uint16(DiscreteStates.CLICK_MAIN);        
%SNF multiclick: 
        if uint16(taskOutput.taskType) == uint16(cursorConstants.TASK_MULTICLICK)
            clickState = uint16(taskOutput.clickTarget); %SNF note: this doesn't match the macro defs in discrete states
        else %it's an instructed click target, we're in hover state, and it's not multiclick
            clickState = uint16(DiscreteStates.CLICK_MAIN); % tag it as clicking. CLICK_MAIN = 1, btw. 
        end 
%end multiclick mod
    end
else % the participant is timing the click either through movement (I think that's what the glove/mouse is) or BCI
    switch clickParameters.clickSource
        case clickConstants.CLICK_TYPE_GLOVE
            if mean(double(gloveData(clickParameters.gloveIndices))) > double(clickParameters.gloveThreshold)
                clickState = uint16(DiscreteStates.CLICK_MAIN);
            end
        case clickConstants.CLICK_TYPE_NEURAL % Closed-loop for multiclick or generic X.1 DoF click task
            % use *stateLikelihoods* not *clickStateLikelihood* for MC: 
            if uint16(taskOutput.taskType) == uint16(cursorConstants.TASK_MULTICLICK)
            % see which clicks are above threshold and make clickState the most likely.
            % Could also return all the clickState values and have the task to decide.
            % Let's go with the largest for now. 
            %%% SNF wonders aloud if we should exclude move from the max calculation
%                 [maxL, maxCS] = max(uint16(decoderOutput.stateLikelihoods)); 
%                 if (maxCS > 1) && (maxL >= clickParameters.hmmClickLikelihoodThreshold)%if the likelihood isn't move AND it's above threshold
%                     clickState = uint16(maxCS); % temporary click state = actual click state
                 [maxL, maxCS] = max(uint16(decoderOutput.stateLikelihoods(CLICK_INDICES))); %SNF: I think Simulink hates "end"
                 if maxL  >= double(clickParameters.hmmClickLikelihoodThreshold)
                     clickState = uint16(maxCS + 1); % temporary click state = actual click state
                else %othersise it's idle 
                    clickState = uint16(DiscreteStates.CLICK_IDLE);
                end
            else % the easy unmodified OG of click decoding: 
                if decoderOutput.clickStateLikelihood >= clickParameters.hmmClickLikelihoodThreshold ...
                        && speed < clickParameters.hmmClickSpeedMax
                    clickState = uint16(DiscreteStates.CLICK_MAIN);
                end
            end
        case clickConstants.CLICK_TYPE_MOUSE
            %% mouse left click is mouseData[4]
            if double(mouseData(4)) > 0
                clickState = uint16(DiscreteStates.CLICK_MAIN);
            end
    end
end

clickStateOut = clickState;
